simulink model "Tut20_SRFlipFlop"  (R2021a)
settings: Solver=FixedStepDiscrete  StartTime=0.0  StopTime=30  FixedStep=1  RelTol=1e-3
libraries: simulink_extras x1
settings Model: Creator=cheta  LastModifiedBy=cheta

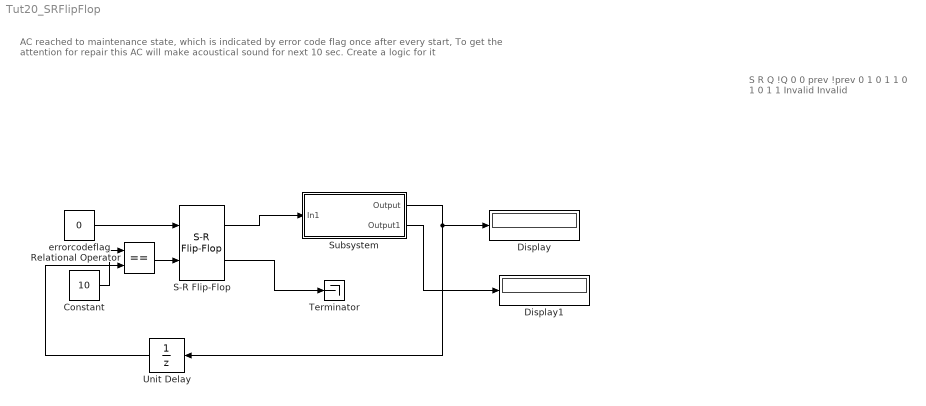
== system Tut20_SRFlipFlop ==
  note: S		R		Q		!Q
      | 0		0		prev		!prev
      | 0		1		0		1
      | 1		0		1		0
      | 1		1		Invalid	Invalid
  note: AC reached to maintenance state, which is indicated by error code flag once after every start,
      | To get the attention for repair this AC will make acoustical sound for next 10 sec.
      |
      | Create a logic for it
  Constant : Constant  Value=10
  Display : Display
  Display1 : Display
  Relational Operator : RelationalOperator  Operator===  OutDataTypeStr=boolean  RndMeth=Simplest
  S-R Flip-Flop : simulink_extras/Flip Flops/S-R Flip-Flop  initial_condition=0
  Subsystem : Subsystem
  Terminator : Terminator
  Unit Delay : UnitDelay  SampleTime=-1  HasFrameUpgradeWarning=on
  errorcodeflag : Constant  Value=0  OutDataTypeStr=boolean
  wires:
  Subsystem/1(Output) -> Unit Delay/1, Display/1
  errorcodeflag/1 -> S-R Flip-Flop/1
  S-R Flip-Flop/1 -> Subsystem/1(In1)
  S-R Flip-Flop/2 -> Terminator/1
  Relational Operator/1 -> S-R Flip-Flop/2
  Constant/1 -> Relational Operator/1
  Unit Delay/1 -> Relational Operator/2
  Subsystem/2(Output1) -> Display1/1

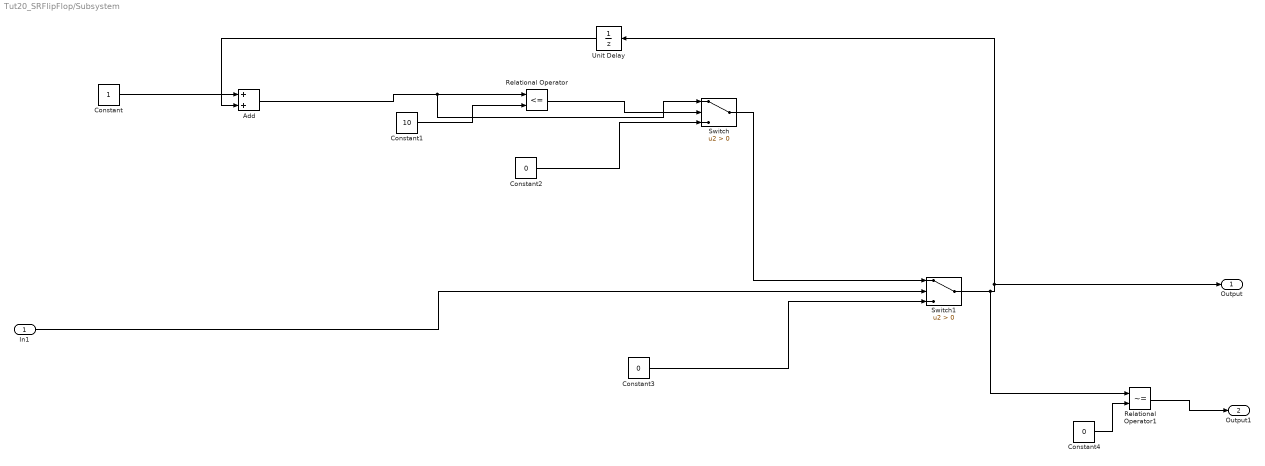
== system Tut20_SRFlipFlop/Subsystem ==
  In1 : Inport
  Add : Sum
  Constant : Constant
  Constant1 : Constant  Value=10
  Constant2 : Constant  Value=0
  Constant3 : Constant  Value=0
  Constant4 : Constant  Value=0
  Relational Operator : RelationalOperator  Operator=<=  OutDataTypeStr=boolean  RndMeth=Simplest
  Relational Operator1 : RelationalOperator  Operator=~=  OutDataTypeStr=boolean  RndMeth=Simplest
  Switch : Switch  Criteria=u2 > Threshold
  Switch1 : Switch  Criteria=u2 > Threshold
  Unit Delay : UnitDelay  SampleTime=-1  HasFrameUpgradeWarning=on
  Output : Outport
  Output1 : Outport  Port=2
  wires:
  Constant/1 -> Add/1
  Add/1 -> Switch/1, Relational Operator/1
  Constant1/1 -> Relational Operator/2
  Relational Operator/1 -> Switch/2
  Constant2/1 -> Switch/3
  Switch/1 -> Switch1/1
  Unit Delay/1 -> Add/2
  In1/1 -> Switch1/2
  Constant3/1 -> Switch1/3
  Switch1/1 -> Relational Operator1/1, Unit Delay/1, Output/1
  Constant4/1 -> Relational Operator1/2
  Relational Operator1/1 -> Output1/1
